simulink model "Ackermann"  (Simulink 5.0)
settings: Solver=ode45  StartTime=0.0  StopTime=10.0  RelTol=1e-3
settings Model: Creator=scaife  LastModifiedBy=scaife  ExtModeAutoUpdateStatusClock=off

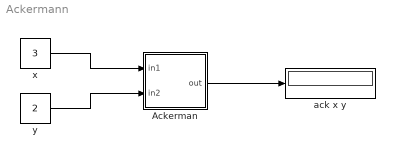
== system Ackermann ==
  Ackerman : Stateflow chart
  ack x y : Display
  x : Constant  Value=3
  y : Constant  Value=2
  wires:
  Ackerman/1(out) -> ack x y/1
  x/1 -> Ackerman/1(in1)
  y/1 -> Ackerman/2(in2)

== stateflow chart Ackerman ==
  state A/
    entry:
    x[1]=in1;
    y[1]=in2;
    mode[1]=1;
    n=1;
  state B/
    entry:
    out=res[n+1];
  state C/
    entry:
    out=-1;
  A -> (junction 6)
  (junction 6) -> (junction 7) : [x[n]>0]
  (default) -> A
  (junction 6) -> (junction 8) : [x[n]==0]
      | {res[n]=y[n]+1;
      |  n--;}
  (junction 9) -> B : [n==0]
  (junction 7) -> (junction 6) : [y[n]==0]
      | {x[n+1]=x[n]-1;
      |  y[n+1]=1;
      |  mode[n+1]=1;
      |  n++;}
  (junction 7) -> (junction 6) : [y[n]>0]
      | {x[n+1]=x[n];
      |  y[n+1]=y[n]-1;
      |  mode[n+1]=2;
      |  n++;}
  (junction 9) -> (junction 6) : [n > 0 & mode[n]==1]
      | {x[n+1]=x[n]-1;
      |  y[n+1]=res[n+1];
      |  mode[n+1]=1;
      |  n++;}
  (junction 9) -> (junction 10) : [n>0 & mode[n]==0]
      | {res[n]=res[n+1];
      |  n--;}
  (junction 10) -> (junction 9)
  (junction 10) -> (junction 9) : [mode[n]>0]
      | {mode[n]--;}
  (junction 8) -> (junction 9)
  (junction 8) -> (junction 9) : [mode[n]>0]
      | {mode[n]--;}
  (junction 6) -> C
  (junction 9) -> C
  (junction 7) -> C
  data: x local uint32 size=10; y local uint32 size=10; n local uint32; mode local uint32 size=10; res local uint32 size=10; in1 input uint32; in2 input uint32; out output uint32
